simulink model "Optimization_Algorithm"  (R2013a)
settings: Solver=ode45  StartTime=0.0  StopTime=10.0  RelTol=1e-3
values from neighbouring files (symbols this model uses):
  fa_differential_ratio = FDR.fa_differential_ratio    [Algorithme_eff.m]    (also in AxelSplitHEVv4_NEDC_18_06_15.mat = 3.72; fa_differential_ratio.mat = 3.72)
  fa_gearbox_ratio = FGR.fa_gearbox_ratio    [Algorithme_eff.m]    (also in AxelSplitHEVv4_NEDC_18_06_15.mat = [0 3.98 2.21 1.47 1.1 0.89 0.75]; fa_gearbox_ratio.mat = [0 3.98 2.21 1.47 1.1 0.89 0.75])
  ra_differential_ratio = RDR.ra_differential_ratio    [Algorithme_eff.m]    (also in AxelSplitHEVv4_NEDC_18_06_15.mat = 10; ra_differential_ratio.mat = 10)
  SP_elec = SPE.SP_elec    [Algorithme_eff.m]    (also in AxelSplitHEVv4_NEDC_18_06_15.mat = [0 150 300 450 600 750 900 1050 1200 1350 1500 1650 ... (81 ; Curve_fitting_elec_eff.m = [SP1 SP2]; Frein_elec.m = ra_electrical_machine_speed(11:21); SP_elec.mat = [0 150 300 450 600 750 900 1050 1200 1350 1500 1650 ... (81 )
  SP_therm = SPT.SP_therm    [Algorithme_eff.m]    (also in AxelSplitHEVv4_NEDC_18_06_15.mat = [800 900 1000 1100 1200 1300 1400 1500 1600 1700 1800 1900 .; Curve_fitting_conso.m = SP(5:end-1); SP_therm.mat = [800 900 1000 1100 1200 1300 1400 1500 1600 1700 1800 1900 .)
  Tab_poly_elec = TPE.Tab_poly_elec    [Algorithme_eff.m]    (also in AxelSplitHEVv4_NEDC_18_06_15.mat = [-3.07907526875e-10 -3.07907526875e-10 -3.07907526875e-10 -3; Curve_fitting_elec_eff.m = [a1_elec;a2_elec]; Tab_poly_elec.mat = [-3.07907526875e-10 -3.07907526875e-10 -3.07907526875e-10 -3)
  Tab_poly_therm = TPT.Tab_poly_therm    [Algorithme_eff.m]    (also in AxelSplitHEVv4_NEDC_18_06_15.mat = [-3.08243117844e-13 -3.21535940734e-13 -3.46421779636e-13 -3; Curve_fitting_conso.m = Tab_poly(5:end-1,:); Tab_poly_therm.mat = [-3.08243117844e-13 -3.21535940734e-13 -3.46421779636e-13 -3)
settings Model: Creator=uidr6416  LastModifiedBy=uidr6416

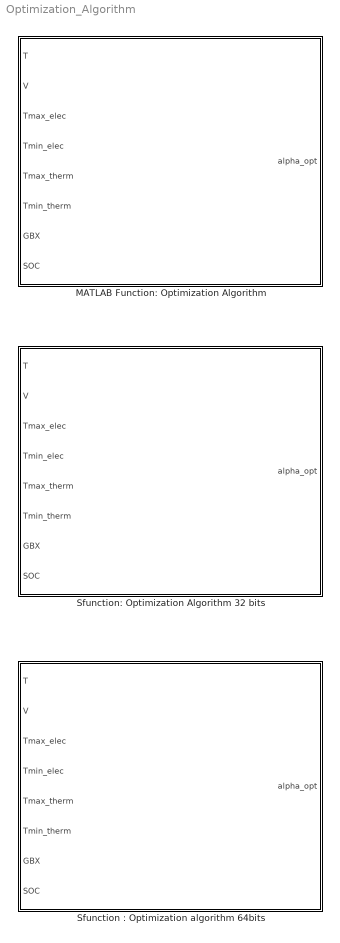
== system Optimization_Algorithm ==
  MATLAB Function: Optimization Algorithm : MATLAB Function  TreatAsAtomicUnit=on
  "Sfunction : Optimization algorithm 64bits" : Subsystem
      mask help: Simulink:masks:GenSFuncDesc_MD
      mask Help: eval('feval(''rtwprivate'',''rtwhelpview'',''rtw_sfcn_block'')');
  Sfunction: Optimization Algorithm 32 bits : Subsystem
      mask help: Simulink:masks:GenSFuncDesc_MD
      mask Help: eval('feval(''rtwprivate'',''rtwhelpview'',''rtw_sfcn_block'')');

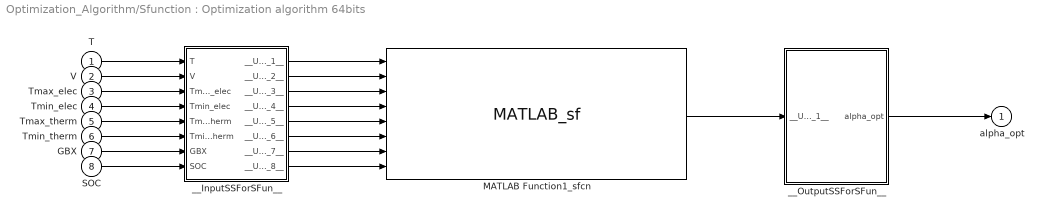
== system Optimization_Algorithm/Sfunction : Optimization algorithm 64bits ==
  T : Inport
  V : Inport  Port=2
  Tmax_elec : Inport  Port=3
  Tmin_elec : Inport  Port=4
  Tmax_therm : Inport  Port=5
  Tmin_therm : Inport  Port=6
  GBX : Inport  Port=7
  SOC : Inport  Port=8
  MATLAB Function1_sfcn : S-Function  FunctionName=MATLAB_sf  SFunctionModules=""  EnableBusSupport=off  mask{rtw_sf_name=MATLAB_sf, showVar=off}
      mask prompts: rtw_sf_name "Simulink:masks:GenSFuncName_MP"; showVar "Simulink:masks:GenSFuncShowModuleList_MP"
      mask help: Simulink:masks:GenSFuncDesc_MD
      mask init:
      | displist = '';
      | if ~strcmp(get_param(gcb, 'FunctionName'), rtw_sf_name);
      |   set_param(gcb, 'FunctionName', rtw_sf_name);
      | end
      | % Check if we are generating code
      | rtw_mode = false;
      | if strcmpi(get_param(bdroot(gcb),'SimulationStatus'),'Initializing')
      | 	rtw_mode = strcmpi(get_param(bdroot(gcb),'BuildingRTWCode'),'on') && ...
      | 		~strcmpi(get_param(bdroot(gcb),'TargetStyle'),'SimulationTarget');
      | end
      | if showVar || rtw_mode
      | 	if exist('rtwsfunc') == 2 | exist('rtwsfunc') == 6
      | 		tmplist = rtwsfunc(rtw_sf_name,gcb);
      | 		tmplist = DAStudio.message('Simulink:masks:GenSFuncListOfModules_IC', tmplist);
      | 	elseif showVar
      | 		tmplist1 = DAStudio.message('Simulink:masks:GenSFuncListOfModules_IC', '');
      |         tmplist2 = DAStudio.message('Simulink:masks:GenSFuncNotLicensed_IC');
      |         tmplist = [tmplist1 tmplist2];
      |  	end
      | end
      | if showVar
      |   displist = tmplist;
      | end
      settings: CopyFcn=|
      | if ~strcmp(get_param(gcb,'Linkstatus'),'none') && ...
      | ~strcmp(get_param(gcb,'Linkstatus'),'implicit')
      |   set_param(gcb,'LinkStatus','none');
      | end
      mask Help: eval('feval(''rtwprivate'',''rtwhelpview'',''rtw_sfcn_block'')');
      mask Display:
      | port_label('input',1,'T');
      | port_label('input',2,'V');
      | port_label('input',3,'Tmax_elec');
      | port_label('input',4,'Tmin_elec');
      | port_label('input',5,'Tmax_therm');
      | port_label('input',6,'Tmin_therm');
      | port_label('input',7,'GBX');
      | port_label('input',8,'SOC');
      | port_label('output',1,'alpha_opt');
  __InputSSForSFun__ : Subsystem
  __OutputSSForSFun__ : Subsystem
  alpha_opt : Outport
  wires:
  T/1 -> __InputSSForSFun__/1(T)
  V/1 -> __InputSSForSFun__/2(V)
  Tmax_elec/1 -> __InputSSForSFun__/3(Tmax_elec)
  Tmin_elec/1 -> __InputSSForSFun__/4(Tmin_elec)
  Tmax_therm/1 -> __InputSSForSFun__/5(Tmax_therm)
  Tmin_therm/1 -> __InputSSForSFun__/6(Tmin_therm)
  GBX/1 -> __InputSSForSFun__/7(GBX)
  SOC/1 -> __InputSSForSFun__/8(SOC)
  __InputSSForSFun__/1(__UniqueOutportName__1__) -> MATLAB Function1_sfcn/1
  __InputSSForSFun__/2(__UniqueOutportName__2__) -> MATLAB Function1_sfcn/2
  __InputSSForSFun__/3(__UniqueOutportName__3__) -> MATLAB Function1_sfcn/3
  __InputSSForSFun__/4(__UniqueOutportName__4__) -> MATLAB Function1_sfcn/4
  __InputSSForSFun__/5(__UniqueOutportName__5__) -> MATLAB Function1_sfcn/5
  __InputSSForSFun__/6(__UniqueOutportName__6__) -> MATLAB Function1_sfcn/6
  __InputSSForSFun__/7(__UniqueOutportName__7__) -> MATLAB Function1_sfcn/7
  __InputSSForSFun__/8(__UniqueOutportName__8__) -> MATLAB Function1_sfcn/8
  MATLAB Function1_sfcn/1 -> __OutputSSForSFun__/1(__UniqueInportName__1__)
  __OutputSSForSFun__/1(alpha_opt) -> alpha_opt/1

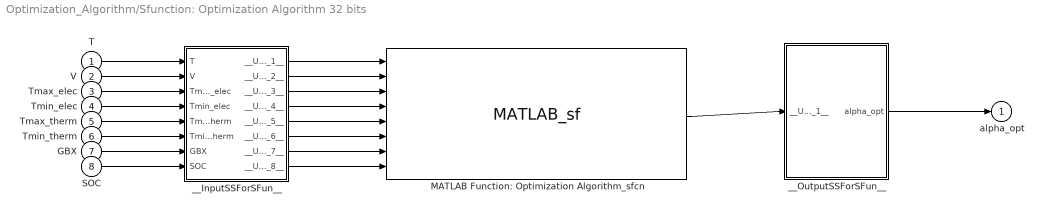
== system Optimization_Algorithm/Sfunction: Optimization Algorithm 32 bits ==
  T : Inport
  V : Inport  Port=2
  Tmax_elec : Inport  Port=3
  Tmin_elec : Inport  Port=4
  Tmax_therm : Inport  Port=5
  Tmin_therm : Inport  Port=6
  GBX : Inport  Port=7
  SOC : Inport  Port=8
  MATLAB Function: Optimization Algorithm_sfcn : S-Function  FunctionName=MATLAB_sf  SFunctionModules=""  EnableBusSupport=off  mask{rtw_sf_name=MATLAB_sf, showVar=off}
      mask prompts: rtw_sf_name "Simulink:masks:GenSFuncName_MP"; showVar "Simulink:masks:GenSFuncShowModuleList_MP"
      mask help: Simulink:masks:GenSFuncDesc_MD
      mask init: same as Optimization_Algorithm/Sfunction : Optimization algorithm 64bits/MATLAB Function1_sfcn
      settings: CopyFcn=|
      | if ~strcmp(get_param(gcb,'Linkstatus'),'none') && ...
      | ~strcmp(get_param(gcb,'Linkstatus'),'implicit')
      |   set_param(gcb,'LinkStatus','none');
      | end
      mask Help: eval('feval(''rtwprivate'',''rtwhelpview'',''rtw_sfcn_block'')');
      mask Display:
      | port_label('input',1,'T');
      | port_label('input',2,'V');
      | port_label('input',3,'Tmax_elec');
      | port_label('input',4,'Tmin_elec');
      | port_label('input',5,'Tmax_therm');
      | port_label('input',6,'Tmin_therm');
      | port_label('input',7,'GBX');
      | port_label('input',8,'SOC');
      | port_label('output',1,'alpha_opt');
  __InputSSForSFun__ : Subsystem
  __OutputSSForSFun__ : Subsystem
  alpha_opt : Outport
  wires:
  T/1 -> __InputSSForSFun__/1(T)
  V/1 -> __InputSSForSFun__/2(V)
  Tmax_elec/1 -> __InputSSForSFun__/3(Tmax_elec)
  Tmin_elec/1 -> __InputSSForSFun__/4(Tmin_elec)
  Tmax_therm/1 -> __InputSSForSFun__/5(Tmax_therm)
  Tmin_therm/1 -> __InputSSForSFun__/6(Tmin_therm)
  GBX/1 -> __InputSSForSFun__/7(GBX)
  SOC/1 -> __InputSSForSFun__/8(SOC)
  __InputSSForSFun__/1(__UniqueOutportName__1__) -> MATLAB Function: Optimization Algorithm_sfcn/1
  __InputSSForSFun__/2(__UniqueOutportName__2__) -> MATLAB Function: Optimization Algorithm_sfcn/2
  __InputSSForSFun__/3(__UniqueOutportName__3__) -> MATLAB Function: Optimization Algorithm_sfcn/3
  __InputSSForSFun__/4(__UniqueOutportName__4__) -> MATLAB Function: Optimization Algorithm_sfcn/4
  __InputSSForSFun__/5(__UniqueOutportName__5__) -> MATLAB Function: Optimization Algorithm_sfcn/5
  __InputSSForSFun__/6(__UniqueOutportName__6__) -> MATLAB Function: Optimization Algorithm_sfcn/6
  __InputSSForSFun__/7(__UniqueOutportName__7__) -> MATLAB Function: Optimization Algorithm_sfcn/7
  __InputSSForSFun__/8(__UniqueOutportName__8__) -> MATLAB Function: Optimization Algorithm_sfcn/8
  MATLAB Function: Optimization Algorithm_sfcn/1 -> __OutputSSForSFun__/1(__UniqueInportName__1__)
  __OutputSSForSFun__/1(alpha_opt) -> alpha_opt/1

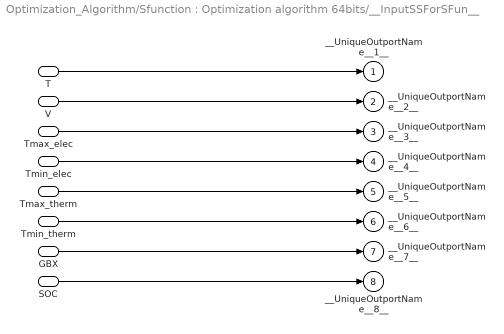
== system Optimization_Algorithm/Sfunction : Optimization algorithm 64bits/__InputSSForSFun__ ==
  T : Inport
  V : Inport  Port=2
  Tmax_elec : Inport  Port=3
  Tmin_elec : Inport  Port=4
  Tmax_therm : Inport  Port=5
  Tmin_therm : Inport  Port=6
  GBX : Inport  Port=7
  SOC : Inport  Port=8
  __UniqueOutportName__1__ : Outport
  __UniqueOutportName__2__ : Outport  Port=2
  __UniqueOutportName__3__ : Outport  Port=3
  __UniqueOutportName__4__ : Outport  Port=4
  __UniqueOutportName__5__ : Outport  Port=5
  __UniqueOutportName__6__ : Outport  Port=6
  __UniqueOutportName__7__ : Outport  Port=7
  __UniqueOutportName__8__ : Outport  Port=8
  wires:
  T/1 -> __UniqueOutportName__1__/1
  V/1 -> __UniqueOutportName__2__/1
  Tmax_elec/1 -> __UniqueOutportName__3__/1
  Tmin_elec/1 -> __UniqueOutportName__4__/1
  Tmax_therm/1 -> __UniqueOutportName__5__/1
  Tmin_therm/1 -> __UniqueOutportName__6__/1
  GBX/1 -> __UniqueOutportName__7__/1
  SOC/1 -> __UniqueOutportName__8__/1

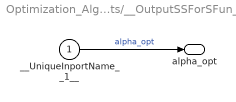
== system Optimization_Algorithm/Sfunction : Optimization algorithm 64bits/__OutputSSForSFun__ ==
  __UniqueInportName__1__ : Inport
  alpha_opt : Outport
  wires:
  __UniqueInportName__1__/1 -> alpha_opt/1  "alpha_opt"

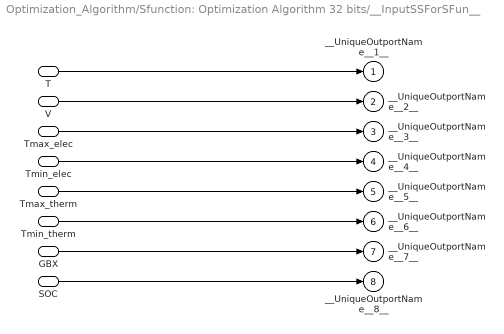
== system Optimization_Algorithm/Sfunction: Optimization Algorithm 32 bits/__InputSSForSFun__ ==
  T : Inport
  V : Inport  Port=2
  Tmax_elec : Inport  Port=3
  Tmin_elec : Inport  Port=4
  Tmax_therm : Inport  Port=5
  Tmin_therm : Inport  Port=6
  GBX : Inport  Port=7
  SOC : Inport  Port=8
  __UniqueOutportName__1__ : Outport
  __UniqueOutportName__2__ : Outport  Port=2
  __UniqueOutportName__3__ : Outport  Port=3
  __UniqueOutportName__4__ : Outport  Port=4
  __UniqueOutportName__5__ : Outport  Port=5
  __UniqueOutportName__6__ : Outport  Port=6
  __UniqueOutportName__7__ : Outport  Port=7
  __UniqueOutportName__8__ : Outport  Port=8
  wires:
  T/1 -> __UniqueOutportName__1__/1
  V/1 -> __UniqueOutportName__2__/1
  Tmax_elec/1 -> __UniqueOutportName__3__/1
  Tmin_elec/1 -> __UniqueOutportName__4__/1
  Tmax_therm/1 -> __UniqueOutportName__5__/1
  Tmin_therm/1 -> __UniqueOutportName__6__/1
  GBX/1 -> __UniqueOutportName__7__/1
  SOC/1 -> __UniqueOutportName__8__/1

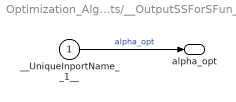
== system Optimization_Algorithm/Sfunction: Optimization Algorithm 32 bits/__OutputSSForSFun__ ==
  __UniqueInportName__1__ : Inport
  alpha_opt : Outport
  wires:
  __UniqueInportName__1__/1 -> alpha_opt/1  "alpha_opt"

== matlab function Optimization_Algorithm/MATLAB Function: Optimization Algorithm ==
  data: T input; alpha_opt output; V input; Tmax_elec input; Tmin_elec input; Tmax_therm input; Tmin_therm input; GBX input; SOC input; SP_elec parameter; SP_therm parameter; fa_differential_ratio parameter; fa_gearbox_ratio parameter; ra_differential_ratio parameter; Tab_poly_therm parameter; Tab_poly_elec parameter
function alpha_opt  = Algorithme_eff(T,V,Tmax_elec,Tmin_elec,Tmax_therm,Tmin_therm,GBX,SOC, SP_elec, SP_therm, fa_differential_ratio, fa_gearbox_ratio, ra_differential_ratio, Tab_poly_therm, Tab_poly_elec)
%%%%%%%%%%%%%%%%%%%%%%%%%%%%%%%%%%%%%%%%%%%%%%%%%%%%%%%%%%%%%%%%%%%%%%%%%%%%%%%%%%%%%%%%%%%%%%%%%%%%
%%%%%%%%%%%% Optimization of torque repartition algorithm (in acceleration phase)%%%%%%%%%%%%%%%%%%% 
%%%%%%%%%%%%%%%%%%%%%%%%%%%%%%%%%%%%%%%%%%%%%%%%%%%%%%%%%%%%%%%%%%%%%%%%%%%%%%%%%%%%%%%%%%%%%%%%%%%%
%%%%%%%%%%          This algorithm minimizes the sum of instantanious consumptions during
%%%%%%%%%%          a prediction horizon . We assume that the torque requested by the
%%%%%%%%%%          driver will always be constant during a prediction horizon that we
%%%%%%%%%%          estimate of 4 seconds (Corresponding N = 400 number of sampling
%%%%%%%%%%          times). The speed is then a slope . Knowing the values of torque and
%%%%%%%%%%          speed , we can express the consumption using the polynoms
%%%%%%%%%%          interpolated from the engines look up tables.
%%%%%%%%%%          Tq_requested = alpha*T_ICE + (1-alpha)*T_elec . 
%%%%%%%%%%          alpha = 0 ===> Pure Electric Mode .  
%%%%%%%%%%          alpha = 1 ===> Pure ICE Mode .
%%%%%%%%%%          The minimization process is a computation of the final criteria with
%%%%%%%%%%          all the possible values of alpha, and then select the minimum . 
%%%%%%%%%%%%%%%%%%%%%%%%%%%%%%%%%%%%%%%%%%%%%%%%%%%%%%%%%%%%%%%%%%%%%%%%%%%%%%%%%%%%%%%%%%%%%%%%%%%%
%%%%%%%%%%%%%%%%%%%%%%%%%%%%%%%%%%%%%%%%%%%%%%%%%%%%%%%%%%%%%%%%%%%%%%%%%%%%%%%%%%%%%%%%%%%%%%%%%%%%
%%%%%%%%%%%%%%%%%%%%%%%%%%%%%%%%%%%%%%%%%%%%%%%%%%%%%%%%%%%%%%%%%%%%%%%%%%%%%%%%%%%%%%%%%%%%%%%%%%%%




%%%%%% Load of necessary variables 
% Done in the model explorer . Necessary variables declared as parameter 

 

%%% Declaration of variables
N = 400; % Determination of Prediction horizon
Sp_elec = zeros(N+1,1) ;  % Elec motor Speed Vector 
Sp_therm = zeros(N+1,1) ; % Therm engine Speed Vector
te = 0.01;  % Sample time 
I_elec = 0 ; % Index Elec 
I_therm = 0 ; % Index Therm
poly_therm = zeros(1,7);  % Polynom coefficient Therm
poly_elec = zeros(1,7);% Polynom coefficient Elec
f = zeros(N,7) ; % Therm criteria  
g = zeros(N,7) ; % Elec  criteria
F = zeros(1,7) ; % Sum of f 
G = zeros(1,7) ; % sum of g 
m = 0 ; % Minimum of consumption 
alpha_opt = 0 ; % alpha optimal 
opt_index = 0 ; % Optimal alpha index 
Sp=zeros(N+1,1); % Speed prediction to the wheels 

Sp(1) = V/(60/(2*(pi))) ;



%% Calcul des bornes de alpha 

alpha_min = max(0,  max( 1 - (Tmax_elec/T) , Tmin_therm/T ) ); 
alpha_max = min(1,min( 1 - (Tmin_elec/T) , Tmax_therm/T ) ); 



if (alpha_max<alpha_min)||(GBX == 0)
    alpha_opt = 0; % Use of electrical if no solutions or gear = 0 
else
    
alpha = alpha_min: 0.01 : alpha_max ; 

S = zeros(1,length(alpha)) ; % Criteria to minimize  

%% Calculus of the predicted speed vector  
for k = 1 : N 
    Sp(k+1) = T*te + Sp(k) ;
end

Sp_elec=Sp*ra_differential_ratio; % Speed in Motor
Sp_therm= Sp*(fa_differential_ratio*fa_gearbox_ratio(GBX+1)); % Speed in engine 


%% Calculus of predicted consumption functions 

T_therm = T/(fa_differential_ratio*fa_gearbox_ratio(GBX+1)) ; % Torque in engine 
T_elec = T/ra_differential_ratio ; % Torque in Motor


for k = 1 : N 
% Determination of corresponding  speed indexes 
I_therm = plus_proche(SP_therm,Sp_therm(k)*(60/(2*(pi)))) ; 
I_elec = plus_proche(SP_elec,Sp_elec(k)*(60/(2*(pi)))) ;

% Extraction of Consumption Polynomials from the tables 
poly_therm = Tab_poly_therm(I_therm,:);
poly_elec = Tab_poly_elec(I_elec,:);

 % Expression of polynomials functions of Alpha
    for p = 1 : 7 
        poly_therm(p) = poly_therm(p)*T_therm^(7-p);
        poly_elec(p) = poly_elec(p)*T_elec^(7-p);
    end
% Kth Polynomial corresponding to Kth speed     
f(k,:) = poly_therm ; 
g(k,:) = -poly_elec ; 

end

% Sum of the polynomials : Final Criteria 
F = sum(f,1); 
G = sum(g,1); 

%% Research of optimal alpha  

 % Calculus of the values of the Criteria for the possible values of alpha 
for k = 1 : length(alpha)
for p = 1 : 7
    S(k) = S(k)   + SOC*F(p)*alpha(k)^(7-p) +  (1-SOC)*G(p)*(1 - alpha(k))^(7-p) ; 
end
end
    
 %Selection of the minimum consumption and the corresponding alpha 
[m,opt_index] = min(S) ; 
alpha_opt = alpha(opt_index) ;

end

end
